simulink model "TRN_V3_CodeGen"  (R2022a)
settings: Solver=FixedStepAuto  StartTime=0.0  StopTime=300  FixedStep=0.04  RelTol=1e-3
PreLoadFcn:
  | % Add DataBus Path
  | addpath(',/TRN');
  | addpath('./MAP/');
  | addpath('./MAP/MAP_DB');
  | addpath('./MAP/DVOF');
  | addpath(genpath(cd));
  | load('BusStructureTRN.mat');
InitFcn:
  | % Add DataBus Path
  | addpath(',/TRN');
  | addpath('./MAP/');
  | addpath('./MAP/MAP_DB');
  | addpath('./MAP/DVOF');
  | addpath(genpath(cd));
  | load('BusStructureTRN.mat');
undefined symbols (not defined in the file or in its folder): Altitude_INS, INSDataNotValid, Latitude_INS, Longitude_INS, RALTValid, TRN, TRNlib
libraries: simulink_extras x33, aerolibconvert2 x6, dspstat3 x3, sharedtransform x2
(part 1 of 3)
settings Model: Creator=HSU  LastModifiedBy=ASCL
settings OptimizationCC: DefaultParameterBehavior=Inlined  UseDivisionForNetSlopeComputation=on  GainParamInheritBuiltInType=on  UseFloatMulNetSlope=on  EnhancedBackFolding=on  PassReuseOutputArgsAs=Individual arguments  ZeroExternalMemoryAtStartup=off  ZeroInternalMemoryAtStartup=off  LifeSpan=Inf  OptimizeBlockOrder=speed  DifferentSizesBufferReuse=on  EfficientTunableParamExpr=on
settings DebuggingCC: ParameterTunabilityLossMsg=error  UnconnectedInputMsg=warning  UnconnectedOutputMsg=warning  UnconnectedLineMsg=warning  SFUnexpectedBacktrackingDiag=warning  SFNoUnconditionalDefaultTransitionDiag=warning
settings HardwareCC: ProdBitPerPointer=32  ProdBitPerSizeT=32  ProdBitPerPtrDiffT=32  ProdLargestAtomicInteger=Long  ProdLargestAtomicFloat=Double  ProdEndianess=BigEndian  ProdWordSize=32  ProdLongLongMode=on  ProdHWDeviceType=Freescale->MPC83xx
settings ModelReferenceCC: ModelReferenceNumInstancesAllowed=Single
settings SFSimCC: SimUserLibraries=MAPd.lib WS2_32.LIB  MATLABDynamicMemAlloc=off
settings SFSimCC: SimCustomHeaderCode=|
  | #include "MAP.h"
  | #include "MAPDATA.h"
  | #include "DVOF.h"
  | #include "userDefined.h"
settings SFSimCC: SimUserSources=|
  | MAP.c
  | DVOF.c
  | userDefined.c
settings RTWCC: SystemTargetFile=ert.tlc  TemplateMakefile=ert_default_tmf  RTWUseSimCustomCode=on  CustomLibrary=MAPd.lib WS2_32.LIB  BuildConfiguration=Debug  DLArmComputeVersion=19.05
settings RTWCC: CustomHeaderCode=|
  | #include "MAP.h"
  | #include "MAPDATA.h"
  | #include "DVOF.h"
  | #include "userDefined.h"
settings RTWCC: CustomSource=|
  | MAP.c
  | DVOF.c
  | userDefined.c
settings CodeAppCC: ForceParamTrailComments=on  IgnoreCustomStorageClasses=off  OperatorAnnotations=on  SimulinkDataObjDesc=on  SFDataObjDesc=on  InsertBlockDesc=on  EnableCustomComments=on
settings ERTTargetCC: TargetLangStandard=C99 (ISO)  GenerateSampleERTMain=on  SuppressErrorStatus=on  SupportAbsoluteTime=off  SupportNonFinite=off  SupportComplex=off  InlinedParameterPlacement=NonHierarchical  ERTCustomFileTemplate=example_file_process.tlc  ERTFilePackagingFormat=CompactWithDataFile  EnableSignedLeftShifts=off  EnableSignedRightShifts=off

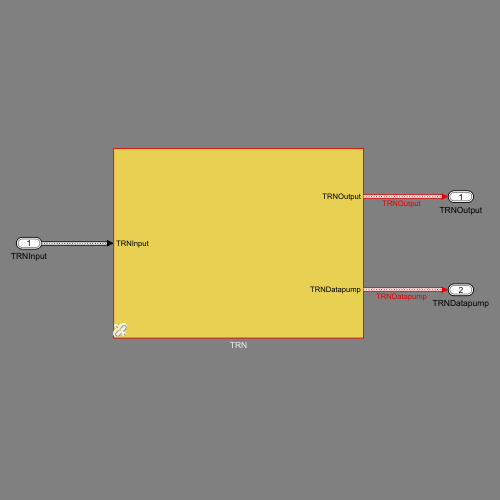
[thumbnail: Simulink's stored preview of the top-level diagram]
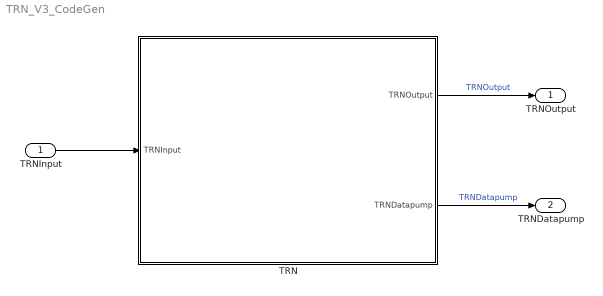
== system TRN_V3_CodeGen ==
  TRNInput : Inport  OutDataTypeStr=Bus: TRNInput  BusOutputAsStruct=on
  TRN : Subsystem  AncestorBlock=TRNlib/TRN
  TRNOutput : Outport  OutDataTypeStr=Bus: TRNOutput  VectorParamsAs1DForOutWhenUnconnected=off  BusOutputAsStruct=on
  TRNDatapump : Outport  Port=2  OutDataTypeStr=Bus: TRNDatapump  VectorParamsAs1DForOutWhenUnconnected=off  BusOutputAsStruct=on
  wires:
  TRN/2(TRNDatapump) -> TRNDatapump/1  "TRNDatapump"
  TRN/1(TRNOutput) -> TRNOutput/1  "TRNOutput"
  TRNInput/1 -> TRN/1(TRNInput)

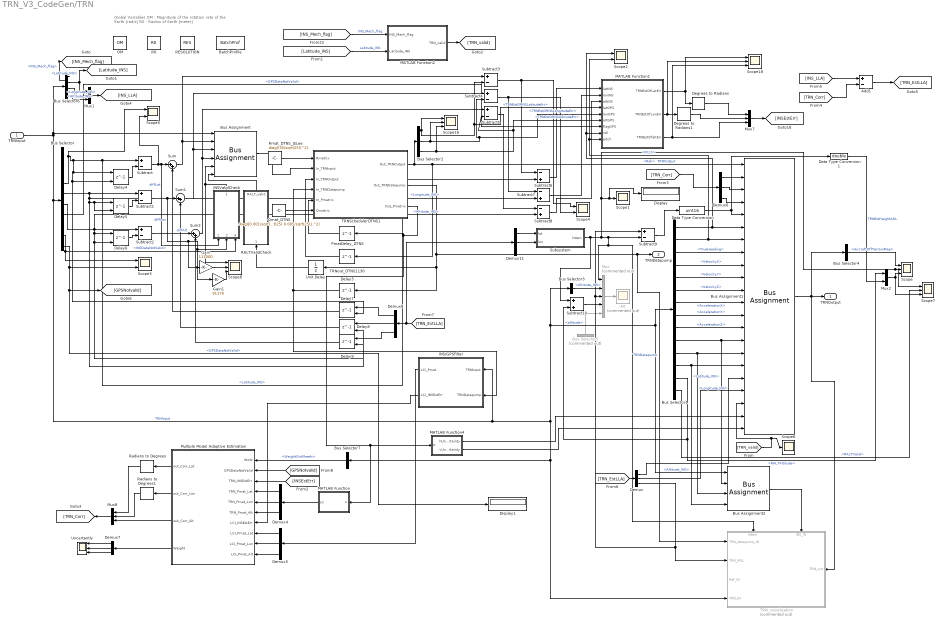
== system TRN_V3_CodeGen/TRN ==
  note: Global Variables
      | OM : Magnitude of the rotation rate of the Earth [rad/s]
      | R0 : Radius of Earth [meter]
  TRNInput : Inport  OutDataTypeStr=Bus: TRNInput
  Add1 : Sum  Inputs=+-
  Alt : Scope  Commented=on
  BatchProfile : DataStoreMemory  DataStoreName=BatchProf  ReadBeforeWriteMsg=warning  WriteAfterWriteMsg=warning  WriteAfterReadMsg=warning  ShowAdditionalParam=off  OutDataTypeStr=double  Dimensions=84200
  Bus Assignment : BusAssignment  AssignedSignals=Latitude_INS,Longitude_INS,Altitude_INS,INSDataNotValid,RALTValid
  Bus Assignment1 : BusAssignment  AssignedSignals=TRNEstOfINSLatitudeErr,TRNEstOfINSLongitudeErr,TRNEstOfINSAltitudeErr,TRNEstHeightAGL,TRN_Roll,TRN_Pitch,TRN_Yaw,TRN_VelocityX,TRN_VelocityY,TRN_VelocityZ,TRN_AccelerationX,TRN_AccelerationY,TRN_AccelerationZ,Latitude_INS,Longitude_INS,Altitude_INS,TRNEstOfLatitude,TRNEstOfLongitude,TRN_valid,TRNHorUncertainty,TRNVerticalUncertainty
  Bus Assignment2 : BusAssignment  AssignedSignals=Latitude_INS,Longitude_INS,Altitude_INS
  Bus Selector : BusSelector  OutputSignals=Latitude_GPS,Longitude_GPS,Altitude_GPS,Latitude_INS,Longitude_INS,Altitude_INS,GPSDataNotValid,RALTValid,INSDataNotValid,GPSDataNotValid
  Bus Selector1 : BusSelector  OutputSignals=Roll,Pitch,TrueHeading,VelocityX,VelocityY,VelocityZ,AccelerationX,AccelerationY,AccelerationZ,Latitude_INS,Longitude_INS,Altitude_INS,RALTAltitude,RALTValid
  Bus Selector2 : BusSelector  OutputSignals=TRNEstOfINSLatitudeErr,TRNEstOfINSLongitudeErr,TRNEstOfINSAltitudeErr
  Bus Selector3 : BusSelector  OutputSignals=Altitude_INS
  Bus Selector4 : BusSelector  OutputSignals=AircraftOffTerrainMap
  Bus Selector5 : BusSelector  Commented=on  OutputSignals=altitude
  Bus Selector6 : BusSelector  OutputSignals=INS_Mech_flag,Latitude_INS,Longitude_INS,Altitude_INS
  Bus Selector7 : BusSelector  OutputSignals=WeightOnWheels
  Data Type Conversion : DataTypeConversion  OutDataTypeStr=uint16  RndMeth=Nearest  SaturateOnIntegerOverflow=off
  Data Type Conversion1 : DataTypeConversion  OutDataTypeStr=double  SaturateOnIntegerOverflow=off  RndMeth=Floor
  Degrees to Radians : simulink_extras/Transformations/Degrees to Radians
  Degrees to Radians1 : simulink_extras/Transformations/Degrees to Radians
  Delay3 : Delay  DelayLength=1  InitialCondition=0
  Delay4 : Delay  DelayLength=1  InitialConditionSource=Input port  InitialCondition=35.2*pi/180
      settings: InputPortMap=u0,p4
  Delay5 : Delay  DelayLength=1  InitialConditionSource=Input port  InitialCondition=35.2*pi/180
      settings: InputPortMap=u0,p4
  Delay6 : Delay  DelayLength=1  InitialConditionSource=Input port  InitialCondition=35.2*pi/180
      settings: InputPortMap=u0,p4
  Delay7 : Delay  DelayLength=1  InitialConditionSource=Input port  InitialCondition=0
      settings: InputPortMap=u0,p4
  Delay8 : Delay  DelayLength=1  InitialConditionSource=Input port  InitialCondition=0
      settings: InputPortMap=u0,p4
  Delay9 : Delay  DelayLength=1  InitialConditionSource=Input port  InitialCondition=0
      settings: InputPortMap=u0,p4
  Demux{,4..8,11} (7 alike) : Demux  Outputs=3
  Display : Display
  Display1 : Display
  Gain : Gain  Gain=111000
  Gain1 : Gain  Gain=91170
  INS/GPSFilter : Subsystem
  INSValidCheck : Subsystem
  MATLAB Function : MATLAB Function  TreatAsAtomicUnit=on
  MATLAB Function1 : MATLAB Function  TreatAsAtomicUnit=on
  MATLAB Function2 : MATLAB Function  TreatAsAtomicUnit=on
  MATLAB Function4 : MATLAB Function  TreatAsAtomicUnit=on
  Multiple Model Adaptive Estimation : MATLAB Function  TreatAsAtomicUnit=on
  Mux : Mux  Commented=on  Inputs=5
  Mux1 : Mux  Inputs=3
  Mux2 : Mux  Inputs=2
  Mux7 : Mux  Inputs=3
  Mux8 : Mux  Inputs=3
  OM : DataStoreMemory  DataStoreName=OM  ReadBeforeWriteMsg=warning  WriteAfterWriteMsg=warning  WriteAfterReadMsg=warning  InitialValue=7.27e-5  ShowAdditionalParam=off
  PmatDelay_DTNS : Delay  DelayLength=1  InitialCondition="diag([0 0 0 0 0 0  10/6378000 10/6378000 13.3 0.0 0.0 0.0 0.00014 0.00014 0.00014 ].^2);"
  Qmat_DTNS : Constant  Value=diag([0.001/sqrt(25) 0.001/sqrt(25) 0.001/sqrt(25) 0.005/sqrt(25) 0.005/sqrt(25) 0.005/sqrt(25)].^2)
  R0 : DataStoreMemory  DataStoreName=R0  ReadBeforeWriteMsg=warning  WriteAfterWriteMsg=warning  WriteAfterReadMsg=warning  InitialValue=6378000  ShowAdditionalParam=off
  RALTValidCheck : Subsystem
  RESOLUTION : DataStoreMemory  DataStoreName=RES  ReadBeforeWriteMsg=warning  WriteAfterWriteMsg=warning  WriteAfterReadMsg=warning  InitialValue=3 * 0.000277777777777777 * 0.0174532925199433  ShowAdditionalParam=off  OutDataTypeStr=double
  Radians to Degrees : simulink_extras/Transformations/Radians to Degrees
  Radians to Degrees1 : simulink_extras/Transformations/Radians to Degrees
  Rmat_DTNS_JSLee : Constant  Value=diag((35/sqrt(25))^2);
  Scope{,7..8,16,18} (5 alike) : Scope  NumInputPorts=3
  Scope1 : Scope
  Scope{2..5} (4 alike) : Scope  NumInputPorts=2
  Scope6 : Scope
  Subsystem : Subsystem
  Subtract{,1..5,9} (7 alike) : Sum  Inputs=+-
  Subtract10 : Sum
  Subtract6 : Sum  Inputs=-+
  Subtract7 : Sum  Inputs=-+
  Subtract8 : Sum  Inputs=-+
  Sum : Sum  Inputs=|++
  Sum1 : Sum  Inputs=|++
  Sum2 : Sum  Inputs=|++
  TRNSchedulerDTNS1 : Stateflow chart  TreatAsAtomicUnit=on
      settings: PortSchema="{\"entries\":[{\"content\":{\"sides\":[{\"content\":{\"connectorIds\":[\"In6\",\"In1\",\"In2\",\"In3\",\"In4\",\"In5\"]},\"type\":\"ConnectorPlacement.EquallySpacedRectSide\",\"uuid\":\"e3a28dc3-1134-4d42-8633-a879e841d02b\"},{\"content\":{\"connectorIds\":[\"Out1\",\"Out2\",\"Out3\"],\"side\":\"RIGHT\"},\"type\":\"ConnectorPlacement.EquallySpacedRectSide\",\"uuid\":\"1aeebddb-d951-4716-a6fa-d3bc83e339ba\"},{\"content\":{\"connectorIds\":[],\"side\":\"TOP\"},\"type\":\"ConnectorPlacement.EquallySpacedRectSide\",\"uuid\":\"d49486c5-974a-4ed9-816b-7cebbe3240fa\"}]},\"type\":\"ConnectorPlacement.EquallySpacedConnector\",\"uuid\":\"19115c55-9321-4bb4-9d4c-d67476a9bc4f\"}],\"packageUris\":[\"http://schema.mathworks.com/mf0/Connector/R2020b\"],\"version\":\"1.0\"}"
  "TRN_visualization " : Subsystem  Commented=on
      settings: PortSchema="{\"entries\":[{\"content\":{\"sides\":[{\"content\":{\"connectorIds\":[\"In1\",\"In2\",\"In3\",\"In4\"]},\"type\":\"ConnectorPlacement.EquallySpacedRectSide\",\"uuid\":\"9b00cbc4-ca0d-429d-9536-38963fe71bc1\"},{\"content\":{\"connectorIds\":[\"In7\"],\"side\":\"RIGHT\"},\"type\":\"ConnectorPlacement.EquallySpacedRectSide\",\"uuid\":\"1db309fb-4b82-499a-a8dc-4a1ba85275fb\"},{\"content\":{\"connectorIds\":[\"In5\",\"In6\"],\"side\":\"TOP\"},\"type\":\"ConnectorPlacement.EquallySpacedRectSide\",\"uuid\":\"7e2d2316-30f0-423f-b46b-636ee0f4a770\"}]},\"type\":\"ConnectorPlacement.EquallySpacedConnector\",\"uuid\":\"aa6e905d-ed4c-45ad-a850-3c33939aad22\"}],\"packageUris\":[\"http://schema.mathworks.com/mf0/Connector/R2020b\"],\"version\":\"1.0\"}"
  TRNout_DTNS1130 : Delay  DelayLength=1  InitialCondition=struct('NavigationMode', false);
  Uncertantly : Scope  NumInputPorts=3
  Unit Delay : UnitDelay  SampleTime=-1  HasFrameUpgradeWarning=on
  TRNOutput : Outport  OutDataTypeStr=Bus: TRNOutput  VectorParamsAs1DForOutWhenUnconnected=off
  TRNDatapump : Outport  Port=2  OutDataTypeStr=Bus: TRNDatapump  VectorParamsAs1DForOutWhenUnconnected=off
  wires:
  Bus Selector2/3 -> Scope16/3, Subtract5/2, MATLAB Function1/6(altGPS)  "<TRNEstOfINSAltitudeErr>"
  Bus Selector2/2 -> Scope16/2, MATLAB Function1/5(lonGPS), Subtract4/2  "<TRNEstOfINSLongitudeErr>"
  Bus Selector2/1 -> MATLAB Function1/4(latGPS), Subtract3/2, Scope16/1  "<TRNEstOfINSLatitudeErr>"
  MATLAB Function4/2(vUncertainty) -> Bus Assignment1/22
  MATLAB Function4/1(hUncertainty) -> Bus Assignment1/21
  Bus Selector/10 -> Display1/1, [GPSNotvalid], Scope3/2  "<GPSDataNotValid>"
  Bus Selector/9 -> INSValidCheck/3(INSDataValid), Scope3/1  "<INSDataNotValid>"
  Bus Selector1/14 -> Scope7/2  "<RALTValid>"
  Mux2/1 -> Scope/3, Scope7/3
  Data Type Conversion1/1 -> Mux2/2  "TRNEstHeightAGL"
  Subsystem/1(hdem) -> Subtract10/1, Subtract9/2, "TRN_visualization "/5(hdem), Mux/1, Scope1/1, Display/1, Scope/2, Scope7/1
  Bus Selector1/13 -> Subtract10/2, Mux2/1  "<RALTAltitude>"
  Bus Selector4/1 -> Scope/1  "<AircraftOffTerrainMap>"
  Subtract10/1 -> Mux/4
  Bus Selector5/1 -> Mux/5  "<altitude>"
  [INS_Mech_flag] -> MATLAB Function2/1(INS_Mech_flag)  "INS_Mech_flag"
  [Latitude_INS] -> MATLAB Function2/2(Latitude_INS)  "Latitude_INS"
  [TRN_valid] -> Scope6/1, Bus Assignment1/20
  MATLAB Function2/1(TRN_valid) -> [TRN_valid]
  Bus Selector6/2 -> [Latitude_INS], Mux1/1  "<Latitude_INS>"
  Bus Selector6/1 -> [INS_Mech_flag]  "<INS_Mech_flag>"
  MATLAB Function/1(yy) -> Demux4/1
  Bus Assignment/1 -> TRNSchedulerDTNS1/1(In_TRNInput)
  Bus Selector/5 -> Delay8/2, Delay5/2, Delay5/1, Subtract7/2, Subtract1/1  "<Longitude_INS>"
  Bus Selector1/3 -> Bus Assignment1/8  "<TrueHeading>"
  Bus Assignment2/1 -> "TRN_visualization "/6(INS_IN)
  Bus Selector1/12 -> Bus Assignment2/4, Bus Assignment1/17  "<Altitude_INS>"
  Bus Selector1/11 -> Bus Assignment2/3, Bus Assignment1/16  "<Longitude_INS>"
  Bus Selector1/10 -> Bus Assignment2/2, Bus Assignment1/15  "<Latitude_INS>"
  Mux/1 -> Alt/1
  Bus Selector3/1 -> Mux/2  "<Altitude_INS>"
  Bus Selector1/9 -> Bus Assignment1/14  "<AccelerationZ>"
  Bus Selector1/8 -> Bus Assignment1/13  "<AccelerationY>"
  Bus Selector1/7 -> Bus Assignment1/12  "<AccelerationX>"
  Bus Selector1/6 -> Bus Assignment1/11  "<VelocityZ>"
  Bus Selector1/5 -> Bus Assignment1/10  "<VelocityY>"
  Bus Selector1/4 -> Bus Assignment1/9  "<VelocityX>"
  Bus Selector1/2 -> Scope2/2, MATLAB Function1/9(pitch), Bus Assignment1/7  "<Pitch>"
  Bus Selector1/1 -> MATLAB Function1/8(roll), Scope2/1, Bus Assignment1/6  "<Roll>"
  TRNInput/1 -> Bus Assignment/1, Bus Selector6/1, Bus Selector/1, INS/GPSFilter/1(TRNInput), Bus Selector1/1, Bus Assignment2/1, Bus Selector3/1, "TRN_visualization "/4(TRN_IN), Bus Selector7/1  "TRNInput"
  TRNSchedulerDTNS1/1(Out_TRNOutput) -> Bus Selector2/1, Bus Assignment1/1, TRNout_DTNS1130/1  "TRNOutput"
  TRNSchedulerDTNS1/2(Out_TRNDatapump) -> Unit Delay/1, Delay3/1, TRNDatapump/1, "TRN_visualization "/1(TRN_datapump_IN)  "TRNDatapump"
  PmatDelay_DTNS/1 -> TRNSchedulerDTNS1/4(In_Pmatrix)
  TRNSchedulerDTNS1/3(Out_Pmatrix) -> PmatDelay_DTNS/1, MATLAB Function4/1(P), MATLAB Function/1(u)
  TRNout_DTNS1130/1 -> TRNSchedulerDTNS1/2(In_TRNOutput)
  Delay3/1 -> TRNSchedulerDTNS1/3(In_TRNDatapump), INS/GPSFilter/2(TRNDatapump)
  Bus Selector/6 -> Delay9/2, Delay6/2, Delay6/1, Subtract8/2, Subtract2/1  "<Altitude_INS>"
  Bus Selector/4 -> Subtract6/2, Subtract/1, Delay4/1, Delay4/2, Delay7/2, Scope5/1  "<Latitude_INS>"
  Delay4/1 -> Subtract/2
  Delay5/1 -> Subtract1/2
  Delay6/1 -> Subtract2/2
  Sum/1 -> Subtract3/1, Bus Assignment/2
  Sum1/1 -> Subtract4/1, Bus Assignment/3
  Sum2/1 -> Subtract5/1, Bus Assignment/4
  Subtract/1 -> INSValidCheck/1(diffLat), Sum/1, Scope5/2  "diffLat"
  Subtract1/1 -> INSValidCheck/2(diffLon), Gain1/1, Gain/1, Sum1/1  "diffLon"
  Subtract4/1 -> Subtract7/1, Scope4/2
  Subtract2/1 -> Sum2/1  "diffAlt"
  Delay7/1 -> Sum/2
  Delay8/1 -> Sum1/2
  Delay9/1 -> Sum2/2
  Bus Assignment1/1 -> TRNOutput/1, "TRN_visualization "/7(TRN_out), Bus Selector4/1
  Subtract9/1 -> Data Type Conversion/1
  Data Type Conversion/1 -> Bus Assignment1/5, Data Type Conversion1/1
  Subtract6/1 -> MATLAB Function1/1(latINS)
  Subtract7/1 -> MATLAB Function1/2(lonINS)
  Subtract8/1 -> MATLAB Function1/3(altINS)
  MATLAB Function1/3(TRNEstOfaltErr) -> Scope18/3, Mux7/3
  MATLAB Function1/2(TRNEstOfLonErr) -> Scope18/2, Degrees to Radians1/1
  MATLAB Function1/1(TRNEstOfLatErr) -> Degrees to Radians/1, Scope18/1
  Bus Selector/7 -> MATLAB Function1/7(flagGPS)  "<GPSDataNotValid>"
  Gain/1 -> Scope8/2
  Gain1/1 -> Scope8/3
  INS/GPSFilter/1(LCI_Pmat) -> Demux5/1
  INS/GPSFilter/2(LCI_INSEstErr) -> Multiple Model Adaptive Estimation/7(LCI_INSEstErr)
  [INSEstErr] -> Multiple Model Adaptive Estimation/3(TRN_INSEstErr)
  Demux4/3 -> Multiple Model Adaptive Estimation/6(TRN_Pmat_Alt)
  Demux4/1 -> Multiple Model Adaptive Estimation/4(TRN_Pmat_Lat)
  Demux4/2 -> Multiple Model Adaptive Estimation/5(TRN_Pmat_Lon)
  Demux5/1 -> Multiple Model Adaptive Estimation/8(LCI_Pmat_Lat)
  Demux5/3 -> Multiple Model Adaptive Estimation/10(LCI_Pmat_Alt)
  Demux5/2 -> Multiple Model Adaptive Estimation/9(LCI_Pmat_Lon)
  Mux8/1 -> [TRN_Corr]
  Multiple Model Adaptive Estimation/1(out_Corr_Lat) -> Radians to Degrees/1
  Multiple Model Adaptive Estimation/2(out_Corr_Lon) -> Radians to Degrees1/1
  Multiple Model Adaptive Estimation/3(out_Corr_Alt) -> Mux8/3
  [TRN_Corr] -> Demux6/1
  Demux6/1 -> Bus Assignment1/2
  Demux6/2 -> Bus Assignment1/3
  Demux6/3 -> Bus Assignment1/4
  Multiple Model Adaptive Estimation/4(Weight) -> Demux7/1
  Demux7/1 -> Uncertantly/1
  Demux7/2 -> Uncertantly/2
  Demux7/3 -> Uncertantly/3
  Degrees to Radians/1 -> Mux7/1
  Degrees to Radians1/1 -> Mux7/2
  Radians to Degrees/1 -> Mux8/1
  Radians to Degrees1/1 -> Mux8/2
  Subtract5/1 -> Subtract8/1
  Subtract3/1 -> Subtract6/1, Scope4/1
  Mux7/1 -> [INSEstErr]
  Rmat_DTNS_JSLee/1 -> TRNSchedulerDTNS1/6(Rmatrix)
  Demux/3 -> "TRN_visualization "/2(TRN_MSL), Mux/3, Subtract9/1
  [TRN_EstLLA] -> Demux11/1, Demux8/1
  Demux8/1 -> Delay7/1
  Demux8/2 -> Delay8/1
  Demux8/3 -> Delay9/1
  Qmat_DTNS/1 -> TRNSchedulerDTNS1/5(Qmatrix)
  Mux1/1 -> [INS_LLA]
  Bus Selector6/3 -> Mux1/2  "<Longitude_INS>"
  Bus Selector6/4 -> Mux1/3  "<Altitude_INS>"
  [INS_LLA] -> Add1/1
  [TRN_Corr] -> Add1/2
  Add1/1 -> [TRN_EstLLA]
  [TRN_EstLLA] -> Demux/1
  Demux/1 -> Bus Assignment1/18
  Demux/2 -> Bus Assignment1/19
  Demux11/1 -> Subsystem/1(lat)
  Demux11/2 -> Subsystem/2(lon)
  [GPSNotvalid] -> Multiple Model Adaptive Estimation/2(GPSDataNotValid)
  RALTValidCheck/1(RALT_valid) -> Bus Assignment/6
  Unit Delay/1 -> RALTValidCheck/1(TRNDatapump)
  INSValidCheck/1(INSDataNotValid) -> Scope8/1, Bus Assignment/5
  Bus Selector7/1 -> Multiple Model Adaptive Estimation/1(WoW)  "<WeightOnWheels>"

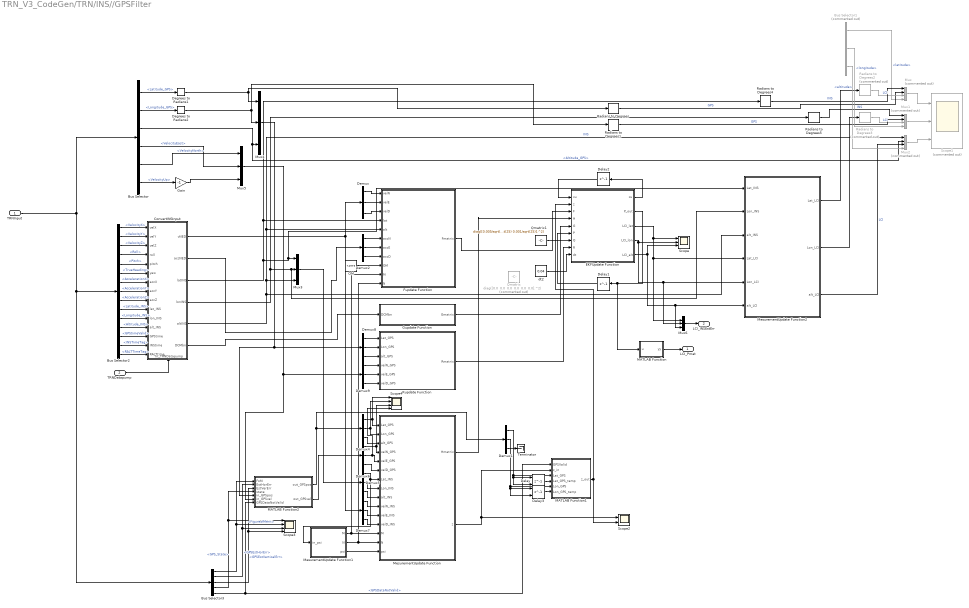
== system TRN_V3_CodeGen/TRN/INS//GPSFilter ==
  TRNInput : Inport
  TRNDatapump : Inport  Port=2
  Bus Selector : BusSelector  OutputSignals=Latitude_GPS,Longitude_GPS,Altitude_GPS,VelocityEast,VelocityNorth,VelocityUp
  Bus Selector1 : BusSelector  Commented=on  OutputSignals=latitude,longitude,altitude
  Bus Selector2 : BusSelector  OutputSignals=VelocityX,VelocityY,VelocityZ,Roll,Pitch,TrueHeading,AccelerationX,AccelerationY,AccelerationZ,Latitude_INS,Longitude_INS,Altitude_INS,GPStimeValid,INSTimeTag,RALTTimeTag
  Bus Selector3 : BusSelector  OutputSignals=FigureofMerit,GPSEstHorErr,GPSEstVerticalErr,GPS_State,GPSDataNotValid
  ConvertINSInput : Subsystem  TreatAsAtomicUnit=on
      settings: PortSchema="{\"entries\":[{\"content\":{\"sides\":[{\"content\":{\"connectorIds\":[\"In1\",\"In2\",\"In3\",\"In4\",\"In5\",\"In6\",\"In7\",\"In8\",\"In9\",\"In10\",\"In11\",\"In12\",\"In13\",\"In14\",\"In15\"]},\"type\":\"ConnectorPlacement.EquallySpacedRectSide\",\"uuid\":\"f8d9ddb6-77a8-494e-a3f5-85bab0322644\"},{\"content\":{\"connectorIds\":[\"Out1\",\"Out2\",\"Out3\",\"Out4\",\"Out5\",\"Out6\"],\"side\":\"RIGHT\"},\"type\":\"ConnectorPlacement.EquallySpacedRectSide\",\"uuid\":\"6d569f5c-c663-4a8e-ac64-f4e4fb828978\"},{\"content\":{\"connectorIds\":[],\"side\":\"TOP\"},\"type\":\"ConnectorPlacement.EquallySpacedRectSide\",\"uuid\":\"3191df82-22b9-436f-88b7-94bbf7c8bdf7\"},{\"content\":{\"connectorIds\":[\"In16\"],\"side\":\"BOTTOM\"},\"type\":\"ConnectorPlacement.EquallySpacedRectSide\",\"uuid\":\"0e180e6a-0c88-4e41-a9aa-7af0a3a32027\"}]},\"type\":\"ConnectorPlacement.EquallySpacedConnector\",\"uuid\":\"a448e351-c7fd-4ddb-9d92-2a19f8cdf805\"}],\"packageUris\":[\"http://schema.mathworks.com/mf0/Connector/R2020b\"],\"version\":\"1.0\"}"
  Degrees to Radians1 : simulink_extras/Transformations/Degrees to Radians
  Degrees to Radians2 : simulink_extras/Transformations/Degrees to Radians
  Delay : Delay  DelayLength=1  InitialConditionSource=Input port
      settings: InputPortMap=u0,p4
  Delay1 : Delay  DelayLength=1  InitialCondition=diag([10/6378000 10/6378000 13.3 0 0 0 0 0 0].^2);
  Delay2 : Delay  DelayLength=1  InitialCondition=[0 0 0 0 0 0 0 0 0]
  Delay3 : Delay  DelayLength=1  InitialConditionSource=Input port
      settings: InputPortMap=u0,p4
  Demux{,1..2,4..9} (9 alike) : Demux  Outputs=3
  EKFUpdate Function : MATLAB Function  TreatAsAtomicUnit=on
  Fupdate Function : MATLAB Function  TreatAsAtomicUnit=on
  Gain : Gain  Gain=-1
  Gupdate Function : MATLAB Function  TreatAsAtomicUnit=on
  MATLAB Function : MATLAB Function  TreatAsAtomicUnit=on
  MATLAB Function1 : MATLAB Function  TreatAsAtomicUnit=on
  MATLAB Function2 : MATLAB Function  TreatAsAtomicUnit=on
  MesurementUpdate Function : MATLAB Function  TreatAsAtomicUnit=on
  MesurementUpdate Function1 : MATLAB Function  TreatAsAtomicUnit=on
  MesurementUpdate Function2 : MATLAB Function  TreatAsAtomicUnit=on
  Mux : Mux  Commented=on
  Mux1 : Mux  Commented=on
  Mux2 : Mux  Commented=on
  Mux{3..6} (4 alike) : Mux  Inputs=3
  OM : Constant  Value=7.27e-5
  Qmatrix : Constant  Commented=on  Value="diag([0.0  0.0  0.0  0.0  0.0  0.0].^2)"
  Qmatrix1 : Constant  Value=diag([0.005/sqrt(25) 0.005/sqrt(25) 0.005/sqrt(25) 0.005/sqrt(25) 0.005/sqrt(25) 0.001/sqrt(25)].^2)
  Radians to Degrees{,1,4..5} (4 alike) : simulink_extras/Transformations/Radians to Degrees
  Radians to Degrees2 : simulink_extras/Transformations/Radians to Degrees  Commented=on
  Radians to Degrees3 : simulink_extras/Transformations/Radians to Degrees  Commented=on
  Rupdate Function : MATLAB Function  TreatAsAtomicUnit=on
  Scope : Scope  NumInputPorts=3
  Scope1 : Scope  Commented=on  NumInputPorts=3
  Scope2 : Scope  NumInputPorts=2
  Scope3 : Scope  NumInputPorts=4
  Scope4 : Scope  NumInputPorts=4
  Terminator : Terminator
  dt2 : Constant  Value=0.04  OutDataTypeStr=double
  LCI_Pmat : Outport
  LCI_INSEstErr : Outport  Port=2
  wires:
  Demux7/3 -> MesurementUpdate Function/12(velD_INS)
  ConvertINSInput/3(latINS) -> Fupdate Function/4(lat), Radians to Degrees4/1, MesurementUpdate Function2/1(Lat_INS), Mux3/1
  MesurementUpdate Function2/2(Lon_LCI) -> Radians to Degrees3/1
  Mux5/1 -> MATLAB Function2/6(in_GPSvel), Demux9/1
  Degrees to Radians2/1 -> Mux4/2, Radians to Degrees1/1
  Demux/1 -> Fupdate Function/1(velN)
  MesurementUpdate Function2/1(Lat_LCI) -> Radians to Degrees2/1
  EKFUpdate Function/4(LCI_lon) -> Mux6/2, MesurementUpdate Function2/5("Lon_LCI "), Scope/2
  Demux9/3 -> Rupdate Function/6(velD_GPS)
  ConvertINSInput/1(vNED) -> Demux7/1, Demux/1
  Demux6/3 -> MesurementUpdate Function/6(velD_GPS)
  Demux2/1 -> Fupdate Function/6(accN)
  Delay1/1 -> EKFUpdate Function/6(P)
  Bus Selector/3 -> Mux2/2, Mux4/3  "<Altitude_GPS>"
  Qmatrix1/1 -> EKFUpdate Function/7(Q)
  EKFUpdate Function/2(P_out) -> MATLAB Function/1(u), Delay1/1
  Demux7/2 -> MesurementUpdate Function/11(velE_INS)
  Demux/2 -> Fupdate Function/2(velE)
  Mux3/1 -> Demux5/1
  OM/1 -> Fupdate Function/9(OM)
  Fupdate Function/1(Fmatrix) -> EKFUpdate Function/3(F)
  dt2/1 -> EKFUpdate Function/9(dt)
  Radians to Degrees3/1 -> Mux1/3  "LCI"
  Demux5/3 -> MesurementUpdate Function/9(alt_INS)
  MesurementUpdate Function/1(Hmatrix) -> EKFUpdate Function/4(H)
  Degrees to Radians1/1 -> Mux4/1, Radians to Degrees/1
  Demux4/2 -> MesurementUpdate Function/2(Lon_GPS), Scope4/2
  Demux8/2 -> Rupdate Function/2(Lon_GPS)
  Bus Selector1/1 -> Mux/4  "<latitude>"
  MesurementUpdate Function2/3(alt_LCI) -> Mux2/3  "LCI"
  Demux8/3 -> Rupdate Function/3(alt_GPS)
  Mux/1 -> Scope1/1
  ConvertINSInput/2(accNED) -> Demux2/1
  Demux9/1 -> Rupdate Function/4(velN_GPS)
  Demux9/2 -> Rupdate Function/5(velE_GPS)
  Radians to Degrees5/1 -> Mux1/1  "INS"
  Demux8/1 -> Rupdate Function/1(Lat_GPS)
  Demux6/1 -> Scope4/3, MesurementUpdate Function/4(velN_GPS)
  Mux2/1 -> Scope1/3
  MesurementUpdate Function/2(z) -> MATLAB Function1/2(z_in), Scope2/1
  Mux1/1 -> Scope1/2
  Demux4/1 -> MesurementUpdate Function/1(Lat_GPS), Scope4/1
  Rupdate Function/1(Rmatrix) -> EKFUpdate Function/8(R)
  Demux/3 -> Fupdate Function/3(velD)
  Demux5/2 -> MesurementUpdate Function/8(Lon_INS)
  Delay2/1 -> EKFUpdate Function/1("xu ")
  Gupdate Function/1(Gmatrix) -> EKFUpdate Function/5(G)
  MesurementUpdate Function1/3(psi) -> MesurementUpdate Function/15(psi)
  EKFUpdate Function/3(LCI_lat) -> Mux6/1, MesurementUpdate Function2/4("Lat_LCI "), Scope/1
  Demux2/3 -> Fupdate Function/8(accD)
  ConvertINSInput/4(lonINS) -> Radians to Degrees5/1, MesurementUpdate Function2/2(Lon_INS), Mux3/2
  Demux5/1 -> MesurementUpdate Function1/1(in_psi), MesurementUpdate Function/7(Lat_INS)
  Demux2/2 -> Fupdate Function/7(accE)
  Demux6/2 -> Scope4/4, MesurementUpdate Function/5(velE_GPS)
  Demux4/3 -> MesurementUpdate Function/3(alt_GPS)
  ConvertINSInput/5(altINS) -> Fupdate Function/5(alt), Mux2/1, Mux3/3, MesurementUpdate Function2/3(alt_INS)  "INS"
  Radians to Degrees/1 -> Mux/2  "GPS"
  Radians to Degrees2/1 -> Mux/3  "LCI"
  EKFUpdate Function/5(LCI_alt) -> Scope/3, Mux6/3, MesurementUpdate Function2/6("alt_LCI ")
  ConvertINSInput/6(DCMbn) -> Gupdate Function/1(DCMbn)
  EKFUpdate Function/1(xu) -> Delay2/1
  Radians to Degrees4/1 -> Mux/1  "INS"
  Radians to Degrees1/1 -> Mux1/2  "GPS"
  Bus Selector1/2 -> Mux1/4  "<longitude>"
  Mux4/1 -> Demux8/1, MATLAB Function2/5(in_GPSpos)
  Demux7/1 -> MesurementUpdate Function/10(velN_INS)
  MesurementUpdate Function1/2(N) -> Fupdate Function/11(N), MesurementUpdate Function/14(N)
  Bus Selector1/3 -> Mux2/4  "<altitude>"
  MesurementUpdate Function1/1(M) -> Fupdate Function/10(M), MesurementUpdate Function/13(M)
  TRNInput/1 -> Bus Selector/1, Bus Selector3/1, Bus Selector2/1
  Bus Selector/1 -> Degrees to Radians1/1  "<Latitude_GPS>"
  Bus Selector/2 -> Degrees to Radians2/1  "<Longitude_GPS>"
  Bus Selector/6 -> Gain/1  "<VelocityUp>"
  Bus Selector/4 -> Mux5/2  "<VelocityEast>"
  Bus Selector/5 -> Mux5/1  "<VelocityNorth>"
  Gain/1 -> Mux5/3
  Bus Selector2/1 -> ConvertINSInput/1(velX)  "<VelocityX>"
  Bus Selector2/2 -> ConvertINSInput/2(velY)  "<VelocityY>"
  Bus Selector2/3 -> ConvertINSInput/3(velZ)  "<VelocityZ>"
  Bus Selector2/4 -> ConvertINSInput/4(roll)  "<Roll>"
  Bus Selector2/5 -> ConvertINSInput/5(pitch)  "<Pitch>"
  Bus Selector2/6 -> ConvertINSInput/6(yaw)  "<TrueHeading>"
  Bus Selector2/7 -> ConvertINSInput/7(accX)  "<AccelerationX>"
  Bus Selector2/8 -> ConvertINSInput/8(accY)  "<AccelerationY>"
  Bus Selector2/9 -> ConvertINSInput/9(accZ)  "<AccelerationZ>"
  Bus Selector2/10 -> ConvertINSInput/10(lat_INS)  "<Latitude_INS>"
  Bus Selector2/11 -> ConvertINSInput/11(lon_INS)  "<Longitude_INS>"
  Bus Selector2/12 -> ConvertINSInput/12(alt_INS)  "<Altitude_INS>"
  MATLAB Function/1(yy) -> LCI_Pmat/1
  Mux6/1 -> LCI_INSEstErr/1
  Bus Selector2/13 -> ConvertINSInput/13(GPStime)  "<GPStimeValid>"
  Bus Selector2/14 -> ConvertINSInput/14(INStime)  "<INSTimeTag>"
  Bus Selector2/15 -> ConvertINSInput/15(RALTtime)  "<RALTTimeTag>"
  TRNDatapump/1 -> ConvertINSInput/16(In_TRNDatapump)
  MATLAB Function1/1(z_out) -> Scope2/2, EKFUpdate Function/2(z)
  Demux1/1 -> Delay/2, Delay/1, MATLAB Function1/3(Lat_GPS)
  Demux1/2 -> Delay3/1, Delay3/2, MATLAB Function1/5(Lon_GPS)
  Delay/1 -> MATLAB Function1/4(Lat_GPS_temp)
  Delay3/1 -> MATLAB Function1/6(Lon_GPS_temp)
  MATLAB Function2/1(out_GPSpos) -> Demux1/1, Demux4/1
  MATLAB Function2/2(out_GPSvel) -> Demux6/1
  Bus Selector3/1 -> Scope3/2, MATLAB Function2/1(FoM)  "<FigureofMerit>"
  Bus Selector3/2 -> Scope3/3, MATLAB Function2/2(EstHorErr)  "<GPSEstHorErr>"
  Bus Selector3/3 -> MATLAB Function2/3(EstVerErr), Scope3/4  "<GPSEstVerticalErr>"
  Bus Selector3/4 -> Scope3/1, MATLAB Function2/4(state)  "<GPS_State>"
  Bus Selector3/5 -> MATLAB Function1/1(GPSValid), MATLAB Function2/7(GPSDataNotValid)  "<GPSDataNotValid>"
  Demux1/3 -> Terminator/1

== system TRN_V3_CodeGen/TRN/INSValidCheck ==
  diffLat : Inport
  diffLon : Inport  Port=2
  INSDataValid : Inport  Port=3
  MATLAB Function5 : MATLAB Function  TreatAsAtomicUnit=on
  delay : Delay  DelayLength=1  InitialCondition=0
  INSDataNotValid : Outport
  wires:
  delay/1 -> MATLAB Function5/4(in_count)
  diffLon/1 -> MATLAB Function5/2(diff_Lon)
  INSDataValid/1 -> MATLAB Function5/3(Valid)
  MATLAB Function5/2(out_count) -> delay/1
  MATLAB Function5/1(NotValid) -> INSDataNotValid/1  "INSDataNotValid"
  diffLat/1 -> MATLAB Function5/1(diff_Lat)

== system TRN_V3_CodeGen/TRN/RALTValidCheck ==
  TRNDatapump : Inport
  Bus Selector7 : BusSelector  OutputSignals=residual
  Data Type Conversion2 : DataTypeConversion  OutDataTypeStr=boolean  SaturateOnIntegerOverflow=off  RndMeth=Floor
  Gain2 : Gain  Gain=3
  MATLAB Function6 : MATLAB Function  TreatAsAtomicUnit=on
  Scope : Scope
  Scope1 : Scope  NumInputPorts=2
  Standard Deviation : dspstat3/Standard Deviation  run=on  directionMode=Entire input  dimension=1  reset_popup=None  roiEnable=off  roiType=Rectangles  roiPortion=Entire ROI  roiOutput=Individual statistics for each ROI  roiFlag=off
      settings: SourceProductBaseCode=DS
  Unit Delay3 : UnitDelay  SampleTime=-1  HasFrameUpgradeWarning=on
  RALT_valid : Outport
  wires:
  Bus Selector7/1 -> Standard Deviation/1, MATLAB Function6/1(residual)  "<residual>"
  Unit Delay3/1 -> MATLAB Function6/3("count ")
  TRNDatapump/1 -> Bus Selector7/1
  MATLAB Function6/2(count) -> Scope1/2, Unit Delay3/1
  Gain2/1 -> Scope/1, MATLAB Function6/2(sigma_3)
  Standard Deviation/1 -> Gain2/1
  MATLAB Function6/1(RALT_valid) -> Scope1/1, Data Type Conversion2/1
  Data Type Conversion2/1 -> RALT_valid/1

== system TRN_V3_CodeGen/TRN/Subsystem ==
  lat : Inport
  lon : Inport  Port=2
  FTGMapCaching : MATLAB Function  TreatAsAtomicUnit=on
  MATLAB Function : MATLAB Function  Commented=on  TreatAsAtomicUnit=on
  hdem : Outport
  wires:
  lat/1 -> FTGMapCaching/1(lat)
  FTGMapCaching/3(hDEM) -> hdem/1
  lon/1 -> FTGMapCaching/2(lon)

== system TRN_V3_CodeGen/TRN/TRNSchedulerDTNS1/AcquisitionCSU ==
  In_TRNInput : Inport  OutDataTypeStr=Bus: TRNInput  PortDimensions=1
  In_TRNDatapump : Inport  Port=2  OutDataTypeStr=Bus: TRNDatapump  PortDimensions=1
  f : TriggerPort  TriggerType=function-call  VariantControl=Variant
      settings: CopyFcn=Stateflow.SLINSF.SimulinkMan.removeBlockPreDeleteFcn  PreDeleteFcn=Stateflow.SLINSF.SimulinkMan.unsafePredeleteFcn
  AcquisitionCSU : Subsystem  TreatAsAtomicUnit=on
  MAD : Outport  VectorParamsAs1DForOutWhenUnconnected=off
  profileCnt : Outport  Port=2  VectorParamsAs1DForOutWhenUnconnected=off
  posUpdate : Outport  Port=3  VectorParamsAs1DForOutWhenUnconnected=off
  residual : Outport  Port=4  VectorParamsAs1DForOutWhenUnconnected=off
  wires:
  In_TRNInput/1 -> AcquisitionCSU/1(In_TRNInput)
  In_TRNDatapump/1 -> AcquisitionCSU/2(In_TRNDatapump)
  AcquisitionCSU/1(MAD) -> MAD/1
  AcquisitionCSU/2(profileCnt) -> profileCnt/1
  AcquisitionCSU/3(posUpdate) -> posUpdate/1
  AcquisitionCSU/4(residual) -> residual/1

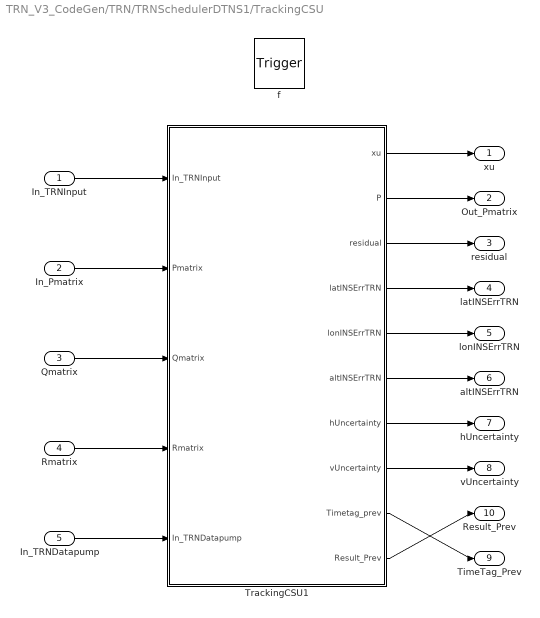
== system TRN_V3_CodeGen/TRN/TRNSchedulerDTNS1/TrackingCSU ==
  In_TRNInput : Inport  OutDataTypeStr=Bus: TRNInput  PortDimensions=1
  In_Pmatrix : Inport  Port=2  OutDataTypeStr=double  PortDimensions=[15 15]
  Qmatrix : Inport  Port=3  OutDataTypeStr=double  PortDimensions=[6 6]
  Rmatrix : Inport  Port=4  OutDataTypeStr=double  PortDimensions=1
  In_TRNDatapump : Inport  Port=5  OutDataTypeStr=Bus: TRNDatapump  PortDimensions=1
  f : TriggerPort  TriggerType=function-call  VariantControl=Variant
      settings: CopyFcn=Stateflow.SLINSF.SimulinkMan.removeBlockPreDeleteFcn  PreDeleteFcn=Stateflow.SLINSF.SimulinkMan.unsafePredeleteFcn
  TrackingCSU1 : Subsystem  TreatAsAtomicUnit=on
  xu : Outport  VectorParamsAs1DForOutWhenUnconnected=off
  Out_Pmatrix : Outport  Port=2  VectorParamsAs1DForOutWhenUnconnected=off
  residual : Outport  Port=3  VectorParamsAs1DForOutWhenUnconnected=off
  latINSErrTRN : Outport  Port=4  VectorParamsAs1DForOutWhenUnconnected=off
  lonINSErrTRN : Outport  Port=5  VectorParamsAs1DForOutWhenUnconnected=off
  altINSErrTRN : Outport  Port=6  VectorParamsAs1DForOutWhenUnconnected=off
  hUncertainty : Outport  Port=7  VectorParamsAs1DForOutWhenUnconnected=off
  vUncertainty : Outport  Port=8  VectorParamsAs1DForOutWhenUnconnected=off
  TimeTag_Prev : Outport  Port=9  VectorParamsAs1DForOutWhenUnconnected=off
  Result_Prev : Outport  Port=10  VectorParamsAs1DForOutWhenUnconnected=off
  wires:
  TrackingCSU1/9(Timetag_prev) -> TimeTag_Prev/1
  TrackingCSU1/10(Result_Prev) -> Result_Prev/1
  TrackingCSU1/3(residual) -> residual/1
  TrackingCSU1/2(P) -> Out_Pmatrix/1
  TrackingCSU1/1(xu) -> xu/1
  In_TRNInput/1 -> TrackingCSU1/1(In_TRNInput)
  In_Pmatrix/1 -> TrackingCSU1/2(Pmatrix)
  Qmatrix/1 -> TrackingCSU1/3(Qmatrix)
  Rmatrix/1 -> TrackingCSU1/4(Rmatrix)
  In_TRNDatapump/1 -> TrackingCSU1/5(In_TRNDatapump)
  TrackingCSU1/4(latINSErrTRN) -> latINSErrTRN/1
  TrackingCSU1/5(lonINSErrTRN) -> lonINSErrTRN/1
  TrackingCSU1/6(altINSErrTRN) -> altINSErrTRN/1
  TrackingCSU1/7(hUncertainty) -> hUncertainty/1
  TrackingCSU1/8(vUncertainty) -> vUncertainty/1

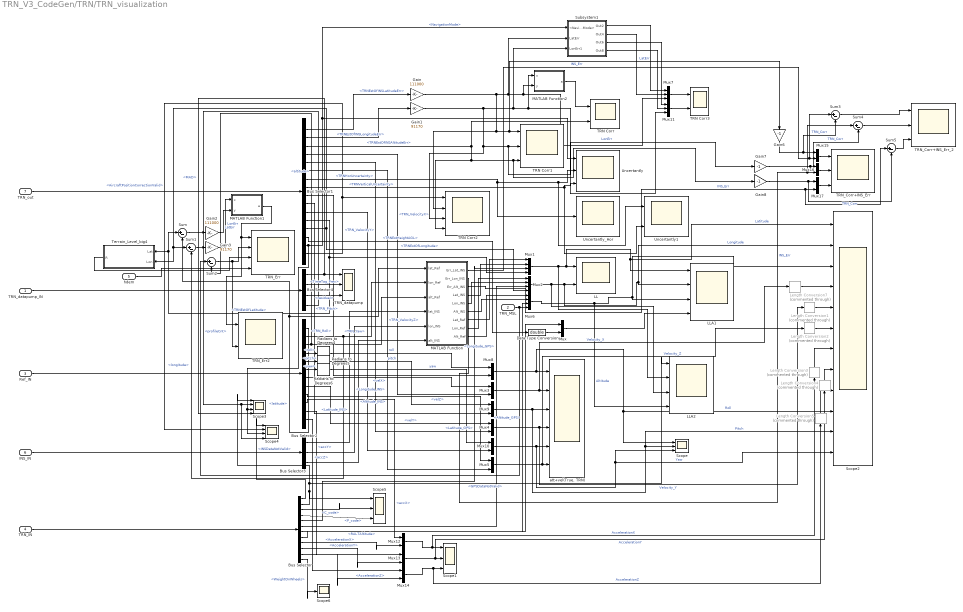
== system TRN_V3_CodeGen/TRN/TRN_visualization  ==
  TRN_datapump_IN : Inport
  TRN_MSL : Inport  Port=2
  Ref_IN : Inport  Port=3
  TRN_IN : Inport  Port=4
  hdem : Inport  Port=5
  INS_IN : Inport  Port=6
  TRN_out : Inport  Port=7
  Bus Selector : BusSelector  OutputSignals=INSDataNotValid,GPSDataNotValid,C_code,P_code,Latitude_GPS,Longitude_GPS,Altitude_GPS,RALTAltitude,AccelerationX,AccelerationY,AccelerationZ,WeightOnWheels
  Bus Selector1 : BusSelector  OutputSignals=TRNEstOfINSLatitudeErr,TRNEstOfINSLongitudeErr,TRNEstOfINSAltitudeErr,TRN_VelocityX,TRN_VelocityY,TRN_VelocityZ,TRNHorUncertainty,TRNVerticalUncertainty,TRN_Roll,TRN_Pitch,TRN_Yaw,TRNEstOfLatitude,TRNEstOfLongitude,TRNEstHeightAGL,NavigationMode,AircraftPositionCorrectionValid
  Bus Selector2 : BusSelector  OutputSignals=latitude,longitude,altitude,roll,pitch,yaw,velX,velY,velZ,accX,accY,accZ
  Bus Selector3 : BusSelector  OutputSignals=Latitude_INS,Longitude_INS,Altitude_INS
  Bus Selector4 : BusSelector  OutputSignals=MAD,TimeTag_Prev,residual,profileCnt
  Data Type Conversion : DataTypeConversion  OutDataTypeStr=double  SaturateOnIntegerOverflow=off  RndMeth=Floor
  Gain : Gain  Gain=111000
  Gain1 : Gain  Gain=91170
  Gain2 : Gain  Gain=111000
  Gain3 : Gain  Gain=91170
  Gain6 : Gain  Gain=-1
  Gain7 : Gain  Gain=-1
  Gain8 : Gain  Gain=-1
  LL : Scope  NumInputPorts=2
  LLA1 : Scope  NumInputPorts=4
  LLA2 : Scope  NumInputPorts=4
  Length Conversion{1..5,7} (6 alike) : aerolibconvert2/Length Conversion  Commented=through  IU=m  OU=ft
  MATLAB Function : MATLAB Function  TreatAsAtomicUnit=on
  MATLAB Function1 : MATLAB Function  TreatAsAtomicUnit=on
  MATLAB Function2 : MATLAB Function  TreatAsAtomicUnit=on
  Mux{,3..5,8..10,12..17} (13 alike) : Mux  Inputs=2
  Mux1 : Mux
  Mux11 : Mux  Inputs=3
  Mux2 : Mux
  Mux6 : Mux
  Mux7 : Mux  Inputs=3
  Radians to Degrees4 : simulink_extras/Transformations/Radians to Degrees
  Radians to Degrees5 : simulink_extras/Transformations/Radians to Degrees
  Radians to Degrees6 : simulink_extras/Transformations/Radians to Degrees
  Scope : Scope  NumInputPorts=3
  Scope1 : Scope  NumInputPorts=3
  Scope2 : Scope  NumInputPorts=12
  Scope3 : Scope  NumInputPorts=4
  Scope4 : Scope  NumInputPorts=4
  Scope5 : Scope  NumInputPorts=3
  Scope6 : Scope
  Subsystem1 : Subsystem
  Sum{,1..5} (6 alike) : Sum  Inputs=|+-
  TRN Corr : Scope  NumInputPorts=2
  TRN Corr1 : Scope  NumInputPorts=3
  TRN Corr2 : Scope  NumInputPorts=4
  TRN Corr3 : Scope  NumInputPorts=2
  TRN_Corr+INS_Err : Scope  NumInputPorts=3
  TRN_Corr+INS_Err_2 : Scope  NumInputPorts=3
  TRN_Err : Scope  NumInputPorts=4
  TRN_Err2 : Scope  NumInputPorts=2
  TRN_datapump : Scope  NumInputPorts=3
  Terrain_Level_big4 : MATLAB Function  TreatAsAtomicUnit=on
  Uncertantly : Scope  NumInputPorts=3
  Uncertantly1 : Scope  NumInputPorts=2
  Uncertantly_Hor : Scope
  "att+vel(True, TRN)" : Scope  NumInputPorts=6
  wires:
  Sum3/1 -> TRN_Corr+INS_Err_2/1
  Sum4/1 -> TRN_Corr+INS_Err_2/2
  Sum5/1 -> TRN_Corr+INS_Err_2/3
  Gain8/1 -> Mux17/1, Sum5/2  "TRN_Corr"
  Gain7/1 -> Mux16/1, Sum4/2  "TRN_Corr"
  Gain6/1 -> Mux15/1, Sum3/2  "TRN_Corr"
  MATLAB Function/3(Err_Alt_INS) -> Mux17/2, Sum5/1  "INS_Err"
  Mux17/1 -> TRN_Corr+INS_Err/3
  MATLAB Function/2(Err_Lon_INS) -> Mux16/2, Sum4/1  "INS_Err"
  Mux16/1 -> TRN_Corr+INS_Err/2
  Mux15/1 -> TRN_Corr+INS_Err/1
  MATLAB Function/1(Err_Lat_INS) -> Mux15/2, Sum3/1  "INS_Err"
  Bus Selector/4 -> Scope5/3  "<P_code>"
  Bus Selector/3 -> Scope5/2  "<C_code>"
  Bus Selector/7 -> Mux6/3  "<Altitude_GPS>"
  Bus Selector/6 -> Mux2/3  "<Longitude_GPS>"
  Bus Selector/5 -> Mux1/3  "<Latitude_GPS>"
  Length Conversion5/1 -> Scope2/9
  Length Conversion4/1 -> Scope2/8
  Length Conversion3/1 -> Scope2/7
  Length Conversion2/1 -> Scope2/6
  Length Conversion1/1 -> Scope2/5
  Length Conversion7/1 -> Scope2/4
  Bus Selector/1 -> Scope4/1  "<INSDataNotValid>"
  Bus Selector4/4 -> Scope3/2, Scope4/4  "<profileCnt>"
  MATLAB Function1/1(a) -> TRN_Err/1, TRN_Err2/1
  Bus Selector/2 -> Scope3/1, LLA2/1, Scope5/1  "<GPSDataNotValid>"
  hdem/1 -> TRN_Err/4
  Terrain_Level_big4/1(R) -> TRN_Err/3
  Bus Selector1/16 -> TRN Corr2/1, Scope4/2  "<AircraftPositionCorrectionValid>"
  Bus Selector1/4 -> Mux3/2  "<TRN_VelocityX>"
  Mux14/1 -> Scope1/3, Length Conversion5/1  "AccelerationZ"
  Bus Selector/11 -> Mux14/2  "<AccelerationZ>"
  Bus Selector2/12 -> Mux14/1  "<accZ>"
  Bus Selector2/11 -> Mux13/1  "<accY>"
  Bus Selector/10 -> Mux13/2  "<AccelerationY>"
  Mux13/1 -> Scope1/2, Length Conversion4/1  "AccelerationY"
  Bus Selector/9 -> Mux12/2  "<AccelerationX>"
  Bus Selector2/10 -> Mux12/1  "<accX>"
  Mux12/1 -> Scope1/1, Length Conversion3/1  "AccelerationX"
  Mux6/1 -> LLA1/3, Scope2/3, LLA2/4  "Altitude"
  Mux/1 -> LLA1/4
  TRN_IN/1 -> Bus Selector/1
  Ref_IN/1 -> Bus Selector2/1
  TRN_out/1 -> Bus Selector1/1
  Gain3/1 -> MATLAB Function1/1(x)  "LonErr"
  Subsystem1/1(Out2) -> Mux7/1
  Mux11/1 -> TRN Corr3/2
  Bus Selector1/8 -> Uncertantly/3, Uncertantly1/2  "<TRNVerticalUncertainty>"
  Bus Selector1/13 -> Sum1/1, Terrain_Level_big4/2(Lon), Mux2/4  "<TRNEstOfLongitude>"
  Radians to Degrees5/1 -> Mux9/1  "pitch"
  Radians to Degrees4/1 -> Mux8/1  "roll"
  Bus Selector2/7 -> Mux3/1  "<velX>"
  MATLAB Function/6(Alt_INS) -> Mux6/2
  Bus Selector1/11 -> Mux10/2  "<TRN_Yaw>"
  Bus Selector1/10 -> Mux9/2  "<TRN_Pitch>"
  Mux3/1 -> "att+vel(True, TRN)"/2, Length Conversion7/1  "Velocity_X"
  Bus Selector1/9 -> Mux8/2  "<TRN_Roll>"
  Bus Selector3/3 -> MATLAB Function/6(alt_INS)  "<Altitude_INS>"
  Bus Selector2/9 -> Mux5/1  "<velZ>"
  Mux4/1 -> "att+vel(True, TRN)"/4, Length Conversion1/1  "Velocity_Y"
  Mux1/1 -> LL/1, LLA1/1, Scope2/1, LLA2/2  "Latitude"
  Mux5/1 -> "att+vel(True, TRN)"/6, Length Conversion2/1  "Velocity_Z"
  Bus Selector2/3 -> MATLAB Function/3(alt_Ref), Sum2/2  "<altitude>"
  Bus Selector1/3 -> TRN Corr2/4, TRN Corr1/3, Gain8/1, TRN Corr/2  "<TRNEstOfINSAltitudeErr>"
  TRN_datapump_IN/1 -> Bus Selector4/1
  Mux2/1 -> LL/2, LLA1/2, Scope2/2, LLA2/3  "Longitude"
  MATLAB Function/9(Alt_Ref) -> Mux6/1
  Gain1/1 -> Mux11/3, MATLAB Function2/1(x), Subsystem1/3(LonErr1), TRN Corr1/2, Gain7/1, TRN Corr2/3  "LonErr"
  MATLAB Function/4(Lat_INS) -> Mux1/2
  Bus Selector3/2 -> MATLAB Function/5(lon_INS)  "<Longitude_INS>"
  Radians to Degrees6/1 -> Mux10/1  "yaw"
  Bus Selector4/2 -> TRN_datapump/2  "<TimeTag_Prev>"
  MATLAB Function/8(Lon_Ref) -> Mux2/1
  Bus Selector2/6 -> Radians to Degrees6/1  "<yaw>"
  MATLAB Function2/1(a) -> TRN Corr/1
  Bus Selector/8 -> Mux/1  "<RALTAltitude>"
  Bus Selector1/15 -> Uncertantly/1, Subsystem1/1(<NavigationMode>), Scope3/3, Scope4/3  "<NavigationMode>"
  Sum2/1 -> TRN_Err/2, TRN_Err2/2
  Bus Selector2/5 -> Radians to Degrees5/1  "<pitch>"
  Mux7/1 -> TRN Corr3/1
  INS_IN/1 -> Bus Selector3/1
  Bus Selector4/1 -> TRN_datapump/1, Scope3/4  "<MAD>"
  Bus Selector1/2 -> Gain1/1  "<TRNEstOfINSLongitudeErr>"
  Bus Selector1/5 -> Mux4/2  "<TRN_VelocityY>"
  Bus Selector3/1 -> MATLAB Function/4(lat_INS)  "<Latitude_INS>"
  Data Type Conversion/1 -> Mux/2
  Subsystem1/3(Out6) -> Mux11/1
  Mux8/1 -> "att+vel(True, TRN)"/1, Scope/1, Scope2/10  "Roll"
  TRN_MSL/1 -> Sum2/1, Mux6/4
  Bus Selector1/14 -> Data Type Conversion/1  "<TRNEstHeightAGL>"
  MATLAB Function/7(Lat_Ref) -> Mux1/1
  Mux9/1 -> "att+vel(True, TRN)"/3, Scope/2, Scope2/11  "Pitch"
  Subsystem1/2(Out4) -> Mux7/2
  Sum1/1 -> Gain3/1
  Bus Selector1/6 -> Mux5/2  "<TRN_VelocityZ>"
  Bus Selector1/1 -> Gain/1  "<TRNEstOfINSLatitudeErr>"
  Bus Selector2/2 -> Sum1/2, MATLAB Function/2(lon_Ref)  "<longitude>"
  Subsystem1/4(Out8) -> Mux11/2
  Gain2/1 -> MATLAB Function1/2(y)  "LatErr"
  Gain/1 -> Mux7/3, MATLAB Function2/2(y), Subsystem1/2(LatErr), TRN Corr1/1, Gain6/1, TRN Corr2/2  "LatErr"
  Bus Selector2/8 -> Mux4/1  "<velY>"
  MATLAB Function/5(Lon_INS) -> Mux2/2
  Bus Selector4/3 -> TRN_datapump/3  "<residual>"
  Bus Selector1/7 -> Uncertantly_Hor/1, Uncertantly/2, Uncertantly1/1  "<TRNHorUncertainty>"
  Sum/1 -> Gain2/1
  Mux10/1 -> "att+vel(True, TRN)"/5, Scope2/12, Scope/3  "Yaw"
  Bus Selector2/1 -> MATLAB Function/1(lat_Ref), Sum/2  "<latitude>"
  Bus Selector2/4 -> Radians to Degrees4/1  "<roll>"
  Bus Selector1/12 -> Sum/1, Terrain_Level_big4/1(Lat), Mux1/4  "<TRNEstOfLatitude>"
  Bus Selector/12 -> Scope6/1  "<WeightOnWheels>"

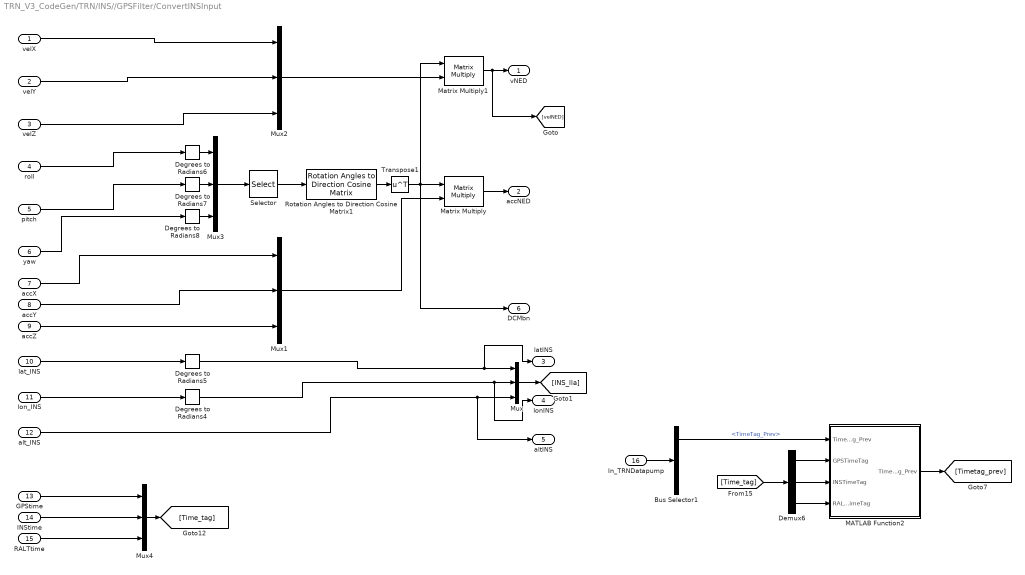
== system TRN_V3_CodeGen/TRN/INS//GPSFilter/ConvertINSInput ==
  velX : Inport
  velY : Inport  Port=2
  velZ : Inport  Port=3
  roll : Inport  Port=4
  pitch : Inport  Port=5
  yaw : Inport  Port=6
  accX : Inport  Port=7
  accY : Inport  Port=8
  accZ : Inport  Port=9
  lat_INS : Inport  Port=10
  lon_INS : Inport  Port=11
  alt_INS : Inport  Port=12
  GPStime : Inport  Port=13
  INStime : Inport  Port=14
  RALTtime : Inport  Port=15
  In_TRNDatapump : Inport  Port=16  OutDataTypeStr=Bus: TRNDatapump  PortDimensions=1
  Bus Selector1 : BusSelector  OutputSignals=TimeTag_Prev,Result_Prev,xu
  Degrees to Radians{4..8} (5 alike) : simulink_extras/Transformations/Degrees to Radians
  Demux6 : Demux  Outputs=3
  MATLAB Function2 : MATLAB Function  TreatAsAtomicUnit=on
  Matrix Multiply : Product  Multiplication=Matrix(*)
  Matrix Multiply1 : Product  Multiplication=Matrix(*)
  Mux{,1..4} (5 alike) : Mux  Inputs=3
  Rotation Angles to Direction Cosine Matrix1 : sharedtransform/Rotation Angles to Direction Cosine Matrix  rotationOrder=ZYX  aMode=aMode
      settings: SourceProductBaseCode=AE
  Selector : Selector  InputPortWidth=3  IndexOptions=Index vector (dialog)  Indices=[3 2 1]  OutputSizes=1
  Transpose1 : Math  Operator=transpose  SignedPower=on
  vNED : Outport  VectorParamsAs1DForOutWhenUnconnected=off
  accNED : Outport  Port=2  VectorParamsAs1DForOutWhenUnconnected=off
  latINS : Outport  Port=3  VectorParamsAs1DForOutWhenUnconnected=off
  lonINS : Outport  Port=4  VectorParamsAs1DForOutWhenUnconnected=off
  altINS : Outport  Port=5  VectorParamsAs1DForOutWhenUnconnected=off
  DCMbn : Outport  Port=6  VectorParamsAs1DForOutWhenUnconnected=off
  wires:
  Degrees to Radians6/1 -> Mux3/1
  Degrees to Radians7/1 -> Mux3/2
  Selector/1 -> Rotation Angles to Direction Cosine Matrix1/1
  Transpose1/1 -> DCMbn/1, Matrix Multiply/1, Matrix Multiply1/1
  Rotation Angles to Direction Cosine Matrix1/1 -> Transpose1/1
  Mux1/1 -> Matrix Multiply/2
  Mux3/1 -> Selector/1
  Matrix Multiply1/1 -> [velNED], vNED/1
  Degrees to Radians8/1 -> Mux3/3
  Matrix Multiply/1 -> accNED/1
  Mux2/1 -> Matrix Multiply1/2
  alt_INS/1 -> altINS/1, Mux/3
  lon_INS/1 -> Degrees to Radians4/1
  accZ/1 -> Mux1/3
  accY/1 -> Mux1/2
  yaw/1 -> Degrees to Radians8/1
  velX/1 -> Mux2/1
  velZ/1 -> Mux2/3
  velY/1 -> Mux2/2
  accX/1 -> Mux1/1
  Degrees to Radians5/1 -> latINS/1, Mux/1
  Degrees to Radians4/1 -> lonINS/1, Mux/2
  pitch/1 -> Degrees to Radians7/1
  lat_INS/1 -> Degrees to Radians5/1
  roll/1 -> Degrees to Radians6/1
  Mux/1 -> [INS_lla]
  Demux6/2 -> MATLAB Function2/3(INSTimeTag)
  In_TRNDatapump/1 -> Bus Selector1/1
  RALTtime/1 -> Mux4/3
  Demux6/3 -> MATLAB Function2/4(RALTTimeTag)
  [Time_tag] -> Demux6/1
  GPStime/1 -> Mux4/1
  Bus Selector1/1 -> MATLAB Function2/1("TimeTag_Prev ")  "<TimeTag_Prev>"
  MATLAB Function2/1(TimeTag_Prev) -> [Timetag_prev]
  INStime/1 -> Mux4/2
  Mux4/1 -> [Time_tag]
  Demux6/1 -> MATLAB Function2/2(GPSTimeTag)

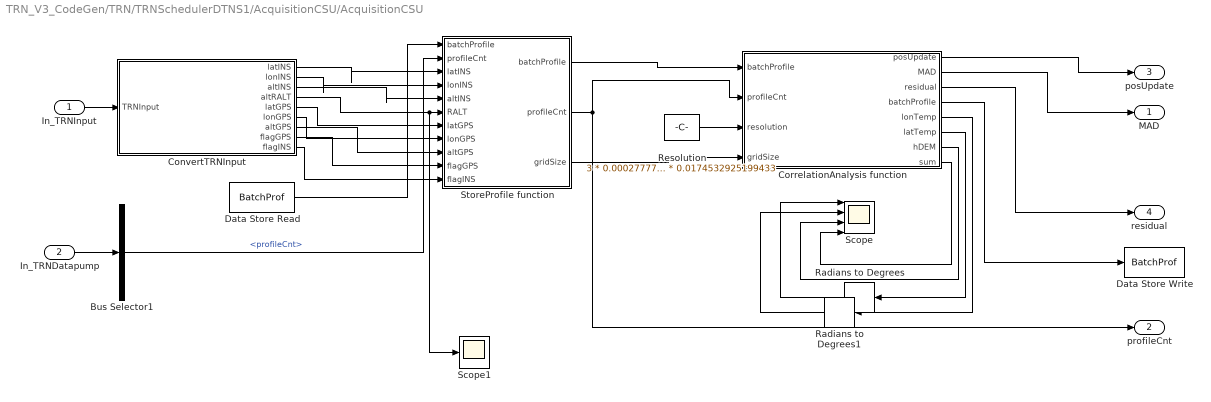
== system TRN_V3_CodeGen/TRN/TRNSchedulerDTNS1/AcquisitionCSU/AcquisitionCSU ==
  In_TRNInput : Inport  OutDataTypeStr=Bus: TRNInput
  In_TRNDatapump : Inport  Port=2  OutDataTypeStr=Bus: TRNDatapump
  Bus Selector1 : BusSelector  OutputSignals=profileCnt
  ConvertTRNInput : Subsystem  TreatAsAtomicUnit=on
  CorrelationAnalysis function : MATLAB Function  TreatAsAtomicUnit=on
  Data Store Read : DataStoreRead  DataStoreName=BatchProf  IndexOptions=Index vector (dialog)  Indices=1  OutputSizes=1
  Data Store Write : DataStoreWrite  DataStoreName=BatchProf  IndexOptions=Index vector (dialog)  Indices=1  OutputSizes=1
  Radians to Degrees : simulink_extras/Transformations/Radians to Degrees
  Radians to Degrees1 : simulink_extras/Transformations/Radians to Degrees
  Resolution : Constant  Value=3 * 0.000277777777777777 * 0.0174532925199433
  Scope : Scope  NumInputPorts=4
  Scope1 : Scope
  StoreProfile function : MATLAB Function  TreatAsAtomicUnit=on
  MAD : Outport  VectorParamsAs1DForOutWhenUnconnected=off
  profileCnt : Outport  Port=2  VectorParamsAs1DForOutWhenUnconnected=off
  posUpdate : Outport  Port=3  VectorParamsAs1DForOutWhenUnconnected=off
  residual : Outport  Port=4  VectorParamsAs1DForOutWhenUnconnected=off
  wires:
  ConvertTRNInput/9(flagINS) -> StoreProfile function/11(flagINS)
  CorrelationAnalysis function/8(sum) -> Scope/4
  CorrelationAnalysis function/7(hDEM) -> Scope/3
  CorrelationAnalysis function/5(lonTemp) -> Radians to Degrees1/1
  CorrelationAnalysis function/6(latTemp) -> Radians to Degrees/1
  In_TRNDatapump/1 -> Bus Selector1/1
  In_TRNInput/1 -> ConvertTRNInput/1(TRNInput)
  Bus Selector1/1 -> StoreProfile function/2("profileCnt ")  "<profileCnt>"
  ConvertTRNInput/1(latINS) -> StoreProfile function/3(latINS)
  ConvertTRNInput/2(lonINS) -> StoreProfile function/4(lonINS)
  ConvertTRNInput/3(altINS) -> StoreProfile function/5(altINS)
  ConvertTRNInput/4(altRALT) -> Scope1/1, StoreProfile function/6(RALT)
  Resolution/1 -> CorrelationAnalysis function/3(resolution)
  StoreProfile function/1(batchProfile) -> CorrelationAnalysis function/1("batchProfile ")
  StoreProfile function/2(profileCnt) -> CorrelationAnalysis function/2(profileCnt), profileCnt/1
  CorrelationAnalysis function/2(MAD) -> MAD/1
  CorrelationAnalysis function/1(posUpdate) -> posUpdate/1
  CorrelationAnalysis function/3(residual) -> residual/1
  StoreProfile function/3(gridSize) -> CorrelationAnalysis function/4(gridSize)
  Data Store Read/1 -> StoreProfile function/1("batchProfile ")
  CorrelationAnalysis function/4(batchProfile) -> Data Store Write/1
  ConvertTRNInput/5(latGPS) -> StoreProfile function/7(latGPS)
  ConvertTRNInput/6(lonGPS) -> StoreProfile function/8(lonGPS)
  ConvertTRNInput/7(altGPS) -> StoreProfile function/9(altGPS)
  ConvertTRNInput/8(flagGPS) -> StoreProfile function/10(flagGPS)
  Radians to Degrees/1 -> Scope/1
  Radians to Degrees1/1 -> Scope/2
